simulink model "nivelTanquePaper"  (R2025a)
settings: Solver=VariableStepAuto  StartTime=0.0  StopTime=30  RelTol=1e-3
libraries: fuzblock x1
settings Model: Creator=Bremdows  LastModifiedBy=Bremdows

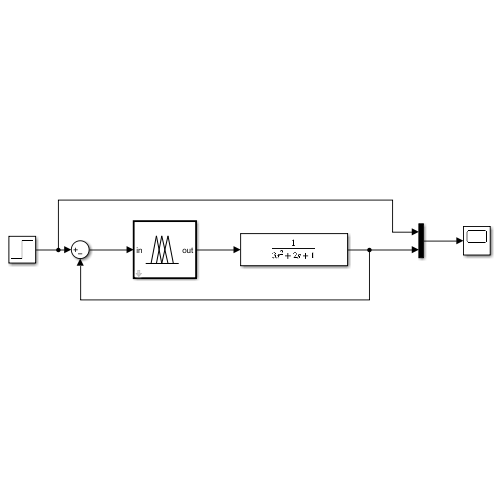
[thumbnail: Simulink's stored preview of the top-level diagram]
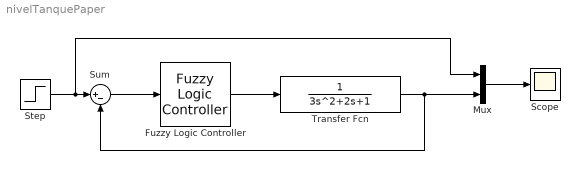
== system nivelTanquePaper ==
  Fuzzy Logic Controller : fuzblock/Fuzzy Logic  Controller  FIS=nivelTanque  OutputSampleNumber=101  DataType=double  UseLookupTable=off  NumBreakpoints=10  FuzzifiedInputs=off  RuleFiringStrengths=off  RuleOutputs=off  AggregatedOutputs=off  SimulateUsing=Interpreted execution  OutOfRangeInputValueMessage=warning  NoRuleFiredMessage=warning  EmptyOutputFuzzySetMessage=warning
  Mux : Mux  Inputs=2
  Scope : Scope
      settings: ActiveDisplayYMinimum=-0.12499999999999997  ActiveDisplayYMaximum=1.125
  Step : Step  Time=0  After=0.5  SampleTime=0
  Sum : Sum  Inputs=|+-
  Transfer Fcn : TransferFcn  Denominator=[3 2 1]
  wires:
  Fuzzy Logic Controller/1 -> Transfer Fcn/1
  Transfer Fcn/1 -> Sum/2, Mux/2
  Step/1 -> Mux/1, Sum/1
  Sum/1 -> Fuzzy Logic Controller/1
  Mux/1 -> Scope/1
